simulink model "hydrocracker_stage7"  (R2025a)
settings: Solver=VariableStepAuto  StartTime=0.0  StopTime=1000  RelTol=1e-3
values from neighbouring files (symbols this model uses):
  A = 5    [hydrocracking.m]
  alpha = 0.5    [hydrocracking.m]
  alpha_r2 = 1.0    (= 1)    [hydrocracking.m]
  CH0 = 1000    [hydrocracking.m]
  CL0 = 0    [hydrocracking.m]
  CM0 = 0    [hydrocracking.m]
  dHrxn = -8e4    (= -80000)    [hydrocracking.m]
  Ea = 8e4    (= 80000)    [hydrocracking.m]
  F_H2in = 0.5    [hydrocracking.m]
  k0 = 1e6    (= 1000000)    [hydrocracking.m]
  nH2_0 = Pset * V_gas / (R*T0)    (= 2.00465078983)    [hydrocracking.m]
  Pset = 1e5    (= 100000)    [hydrocracking.m]
  R = 8.314    [hydrocracking.m]
  rhoCp = 4.0e6    (= 4000000)    [hydrocracking.m]
  T0 = 600    [hydrocracking.m]
  T_cool = 550    [hydrocracking.m]
  tau = 0.5    [hydrocracking.m]
  Tset = 600    [hydrocracking.m]
  U = 500    [hydrocracking.m]
  V_gas = 0.1    [hydrocracking.m]
  V_liq = 1.0    (= 1)    [hydrocracking.m]
libraries: slpidlib x2
settings Model: Creator=brown  LastModifiedBy=brown

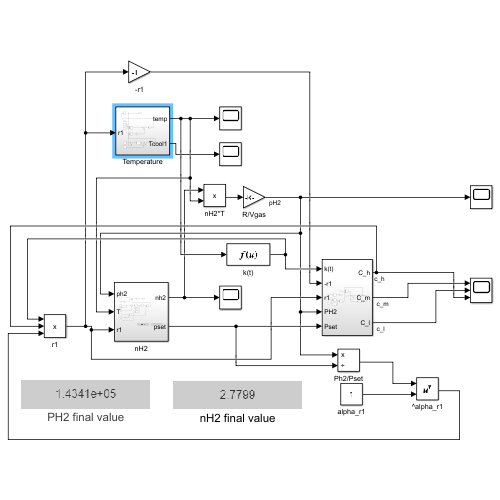
[thumbnail: Simulink's stored preview of the top-level diagram]
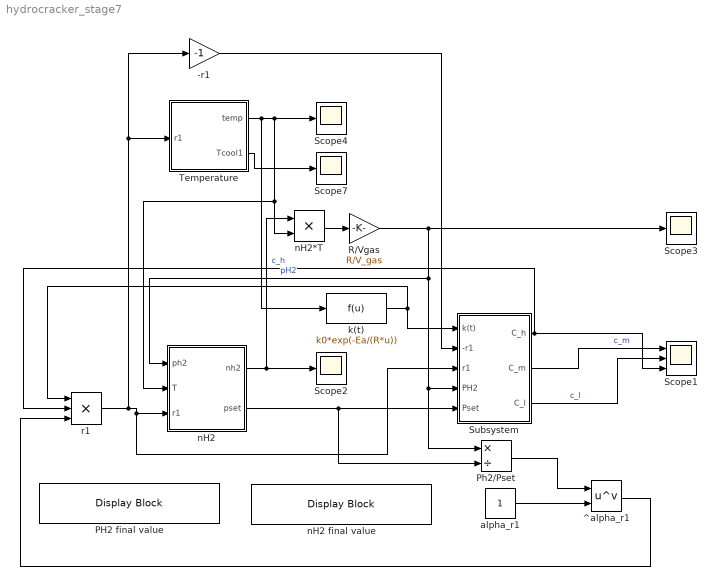
== system hydrocracker_stage7 ==
  -r1 : Gain  Gain=-1
  PH2 final value : DisplayBlock  Description=PH2 final value  LabelPosition=Hide  Transparency=1  GridColor=[0.502, 0.502, 0.502]
      settings: AttributesFormatString=%<Description>
  Ph2/Pset : Product  Inputs=*/
  R/Vgas : Gain  Gain=R/V_gas
  Scope1 : Scope  NumInputPorts=3
      settings: ActiveDisplayYMinimum=-163.95249166903488  ActiveDisplayYMaximum=1598.0751597626968
  Scope{2..4,7} (4 alike) : Scope
      Scope2 settings: ActiveDisplayYMinimum=-0.89806097221704873  ActiveDisplayYMaximum=6.0019022834382847  DataLoggingVariableName=ScopeData2
      Scope3 settings: ActiveDisplayYMinimum=-14020.662869162879  ActiveDisplayYMaximum=16737.974545965073  DataLoggingVariableName=ScopeData3
      Scope4 settings: ActiveDisplayYMinimum=580.56684447993848  ActiveDisplayYMaximum=662.48239747008381  DataLoggingVariableName=ScopeData4
      Scope7 settings: ActiveDisplayYMinimum=520.31544213629388  ActiveDisplayYMaximum=544.27149165677986  DataLoggingVariableName=ScopeData7
  Subsystem : Subsystem
  Temperature : Subsystem
  ^alpha_r1 : Math  Operator=pow
  alpha_r1 : Constant
  k(t) : Fcn  Expr=k0*exp(-Ea/(R*u))
  nH2 : Subsystem
  nH2 final value : DisplayBlock  LabelPosition=Hide  Transparency=1  GridColor=[0.502, 0.502, 0.502]
  nH2*T : Product
  r1 : Product  Inputs=3
  wires:
  k(t)/1 -> r1/1, Subsystem/1(k(t))
  nH2/1(nh2) -> nH2*T/1, Scope2/1
  r1/1 -> Subsystem/3(r1), nH2/3(r1), Temperature/1(r1), -r1/1
  R/Vgas/1 -> Scope3/1, Ph2/Pset/1, Subsystem/4(PH2), nH2/1(ph2)  "pH2"
  Temperature/2(Tcool1) -> Scope7/1
  Temperature/1(temp) -> k(t)/1, nH2/2(T), nH2*T/2, Scope4/1
  -r1/1 -> Subsystem/2(-r1)
  nH2/2(pset) -> Ph2/Pset/2, Subsystem/5(Pset)
  Subsystem/1(C_h) -> Scope1/3, r1/2  "c_h"
  Subsystem/2(C_m) -> Scope1/1  "c_m"
  Subsystem/3(C_l) -> Scope1/2  "c_l"
  Ph2/Pset/1 -> ^alpha_r1/1
  alpha_r1/1 -> ^alpha_r1/2
  ^alpha_r1/1 -> r1/3
  nH2*T/1 -> R/Vgas/1

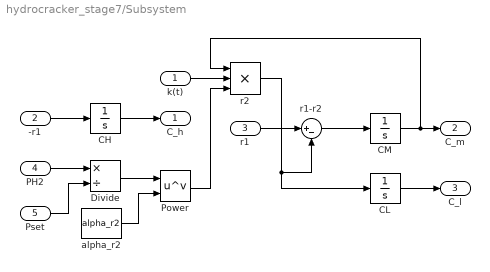
== system hydrocracker_stage7/Subsystem ==
  k(t) : Inport
  -r1 : Inport  Port=2
  r1 : Inport  Port=3
  PH2 : Inport  Port=4
  Pset : Inport  Port=5
  CH : Integrator  InitialCondition=CH0
  CL : Integrator  InitialCondition=CL0
  CM : Integrator  InitialCondition=CM0
  Divide : Product  Inputs=*/
  Power : Math  Operator=pow
  alpha_r2 : Constant  Value=alpha_r2
  r1-r2 : Sum  Inputs=|+-
  r2 : Product  Inputs=3
  C_h : Outport
  C_m : Outport  Port=2
  C_l : Outport  Port=3
  wires:
  r1/1 -> r1-r2/1
  Pset/1 -> Divide/2
  -r1/1 -> CH/1
  PH2/1 -> Divide/1
  Power/1 -> r2/3
  CM/1 -> r2/1, C_m/1
  Divide/1 -> Power/1
  CH/1 -> C_h/1
  r2/1 -> CL/1, r1-r2/2
  alpha_r2/1 -> Power/2
  k(t)/1 -> r2/2
  CL/1 -> C_l/1
  r1-r2/1 -> CM/1

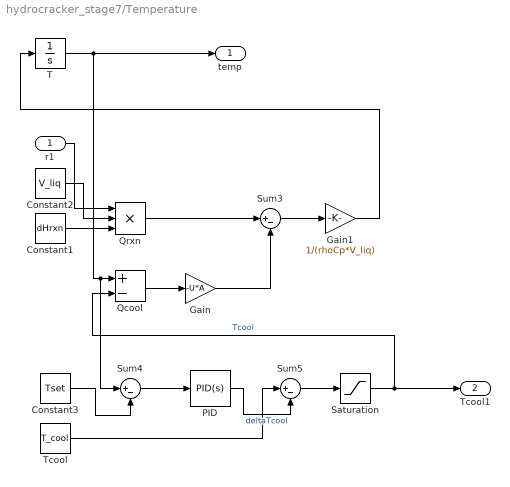
== system hydrocracker_stage7/Temperature ==
  r1 : Inport
  Constant1 : Constant  Value=dHrxn
  Constant2 : Constant  Value=V_liq
  Constant3 : Constant  Value=Tset
  Gain : Gain  Gain=-U*A
  Gain1 : Gain  Gain=1/(rhoCp*V_liq)
  PID : slpidlib/PID Controller  Controller=PID  Form=Parallel  TimeDomain=Continuous-time  UseExternalTs=off  SampleTime=-1  IntegratorMethod=Forward Euler  FilterMethod=Forward Euler  ControllerParametersSource=internal  P=0.5  I=0.001  UseKiTs=off  D=1  UseExternalDerivativeSource=off  N=100  UseFilter=on  TunerSelectOption=Transfer Function Based (PID Tuner App)  InitialConditionSource=internal  InitialConditionForIntegrator=0  InitialConditionForFilter=0  DifferentiatorICPrevScaledInput=0  ExternalReset=none  TrackingMode=off  Kt=1  LimitOutput=on  SatLimitsSource=internal  UpperSaturationLimit=inf  LowerSaturationLimit=0  LinearizeAsGain=on  AntiWindupMode=none  Kb=1  LimitIntegrator=off  UpperIntegratorSaturationLimit=inf  LowerIntegratorSaturationLimit=-inf  POutMin=[]  POutMax=[]  IOutMin=[]  IOutMax=[]  DOutMin=[]  DOutMax=[]  NOutMin=[]  NOutMax=[]  SumOutMin=[]  SumOutMax=[]  SaturationOutMin=[]  SaturationOutMax=[]  PParamMin=[]  PParamMax=[]  IParamMin=[]  IParamMax=[]  DParamMin=[]  DParamMax=[]  NParamMin=[]  NParamMax=[]  KbParamMin=[]  KbParamMax=[]  KtParamMin=[]  KtParamMax=[]  KbOutMin=[]  KbOutMax=[]  KtOutMin=[]  KtOutMax=[]  IntegratorOutMin=[]  IntegratorOutMax=[]  FilterOutMin=[]  FilterOutMax=[]  SumI1OutMin=[]  SumI1OutMax=[]  SumI2OutMin=[]  SumI2OutMax=[]  SumI3OutMin=[]  SumI3OutMax=[]  SumI4OutMin=[]  SumI4OutMax=[]  SumDOutMin=[]  SumDOutMax=[]  DifferentiatorOutMin=[]  DifferentiatorOutMax=[]  FilterDiffOutCoefMin=[]  FilterDiffOutCoefMax=[]  ReciprocalOutMin=[]  ReciprocalOutMax=[]  SumDenOutMin=[]  SumDenOutMax=[]  SumNumOutMin=[]  SumNumOutMax=[]  DivideOutMin=[]  DivideOutMax=[]  UdiffTsProdOutMin=[]  UdiffTsProdOutMax=[]  NTsProdOutMin=[]  NTsProdOutMax=[]  UintegralTsProdOutMin=[]  UintegralTsProdOutMax=[]  UngainTsProdOutMin=[]  UngainTsProdOutMax=[]  ClampingZeroOutDataTypeStr=Inherit: Inherit via back propagation  ClampingZeroOutMin=[]  ClampingZeroOutMax=[]  FilterDenConstantOutDataTypeStr=Inherit: Inherit via back propagation  FilterDenConstantOutMin=[]  FilterDenConstantOutMax=[]  PCopyOutDataTypeStr=Inherit: Inherit via back propagation  PCopyOutMin=[]  PCopyOutMax=[]  NCopyOutDataTypeStr=Inherit: Inherit via back propagation  NCopyOutMin=[]  NCopyOutMax=[]  IntegratorContinuousStateAttributes=''  IntegratorStateMustResolveToSignalObject=off  IntegratorRTWStateStorageClass=Auto  FilterContinuousStateAttributes=''  FilterStateMustResolveToSignalObject=off  FilterRTWStateStorageClass=Auto  ParallelPVariant=InternalParameters  IdealPVariant=Disabled  IVariant=InternalParameters  DVariant=InternalParameters  IntegratorVariant=Continuous  SatVariant=Enabled  AWVariant=Passthrough  PCopyVariant=Disabled  TRVariant=Disabled  FdbkBlocksVariant=Forward  IdealPFdbkVariant=Disabled  SatFdbkVariant=Disabled  DerivativeFilterVariant=ContFilter  NVariant=InternalParameters  NCopyVariant=Disabled  FilterICVariant=InternalICsFilter  IntegratorICVariant=InternalICs  ExternalResetVariant=Disabled  TRSumVariant=Passthrough  SumFdbkVariant=Disabled  SumVariant=Sum_PID  TsampFilterVariant=InternalTs  TsampNgainVariant=Passthrough  TsampIntegralVariant=Disabled_SignalSpec  ExternalSaturationOutDataTypeStr=Inherit: Same as second input  DerivativeSourceVariant=ErrorSignal  PreIntVariant=InternalPreInt
  Qcool : Sum  Inputs=+-
  Qrxn : Product  Inputs=3
  Saturation : Saturate  UpperLimit=600  LowerLimit=350
  Sum3 : Sum  Inputs=|+-
  Sum4 : Sum  Inputs=|+-
  Sum5 : Sum  Inputs=|+-
  T : Integrator  InitialCondition=T0
  Tcool : Constant  Value=T_cool
  temp : Outport
  Tcool1 : Outport  Port=2
  wires:
  Sum5/1 -> Saturation/1
  Saturation/1 -> Tcool1/1, Qcool/2  "Tcool"
  Sum3/1 -> Gain1/1
  Gain1/1 -> T/1
  Sum4/1 -> PID/1
  Constant1/1 -> Qrxn/3
  Constant2/1 -> Qrxn/2
  Tcool/1 -> Sum5/1
  Qcool/1 -> Gain/1
  Gain/1 -> Sum3/2
  PID/1 -> Sum5/2  "deltaTcool"
  Qrxn/1 -> Sum3/1
  T/1 -> Sum4/1, Qcool/1, temp/1
  r1/1 -> Qrxn/1
  Constant3/1 -> Sum4/2

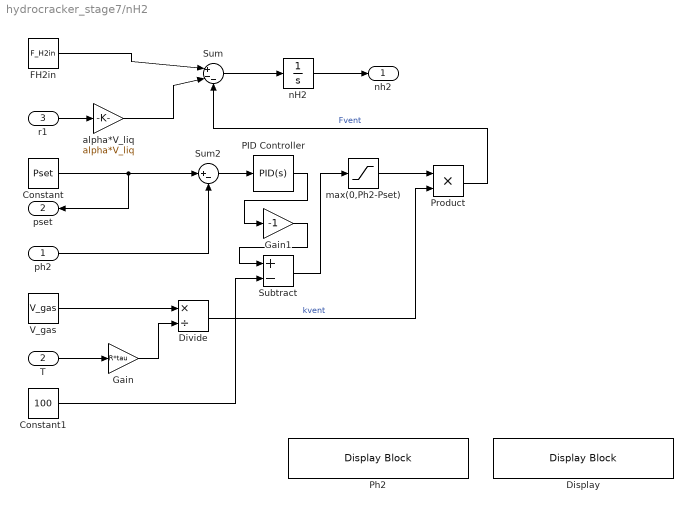
== system hydrocracker_stage7/nH2 ==
  ph2 : Inport
  T : Inport  Port=2
  r1 : Inport  Port=3
  Constant : Constant  Value=Pset
  Constant1 : Constant  Value=100
  Display : DisplayBlock  Description=Fvent  LabelPosition=Hide  Transparency=1  GridColor=[0.502, 0.502, 0.502]
      settings: AttributesFormatString=%<Description>
  Divide : Product  Inputs=*/
  FH2in : Constant  Value=F_H2in
  Gain : Gain  Gain=R*tau
  Gain1 : Gain  Gain=-1
  PID Controller : slpidlib/PID Controller  Controller=PID  Form=Parallel  TimeDomain=Continuous-time  UseExternalTs=off  SampleTime=-1  IntegratorMethod=Forward Euler  FilterMethod=Forward Euler  ControllerParametersSource=internal  P=2e-3  I=2e-4  UseKiTs=off  D=0  UseExternalDerivativeSource=off  N=100  UseFilter=on  TunerSelectOption=Transfer Function Based (PID Tuner App)  InitialConditionSource=internal  InitialConditionForIntegrator=0  InitialConditionForFilter=0  DifferentiatorICPrevScaledInput=0  ExternalReset=none  TrackingMode=off  Kt=1  LimitOutput=on  SatLimitsSource=internal  UpperSaturationLimit=inf  LowerSaturationLimit=0  LinearizeAsGain=on  AntiWindupMode=none  Kb=1  LimitIntegrator=off  UpperIntegratorSaturationLimit=inf  LowerIntegratorSaturationLimit=-inf  POutMin=[]  POutMax=[]  IOutMin=[]  IOutMax=[]  DOutMin=[]  DOutMax=[]  NOutMin=[]  NOutMax=[]  SumOutMin=[]  SumOutMax=[]  SaturationOutMin=[]  SaturationOutMax=[]  PParamMin=[]  PParamMax=[]  IParamMin=[]  IParamMax=[]  DParamMin=[]  DParamMax=[]  NParamMin=[]  NParamMax=[]  KbParamMin=[]  KbParamMax=[]  KtParamMin=[]  KtParamMax=[]  KbOutMin=[]  KbOutMax=[]  KtOutMin=[]  KtOutMax=[]  IntegratorOutMin=[]  IntegratorOutMax=[]  FilterOutMin=[]  FilterOutMax=[]  SumI1OutMin=[]  SumI1OutMax=[]  SumI2OutMin=[]  SumI2OutMax=[]  SumI3OutMin=[]  SumI3OutMax=[]  SumI4OutMin=[]  SumI4OutMax=[]  SumDOutMin=[]  SumDOutMax=[]  DifferentiatorOutMin=[]  DifferentiatorOutMax=[]  FilterDiffOutCoefMin=[]  FilterDiffOutCoefMax=[]  ReciprocalOutMin=[]  ReciprocalOutMax=[]  SumDenOutMin=[]  SumDenOutMax=[]  SumNumOutMin=[]  SumNumOutMax=[]  DivideOutMin=[]  DivideOutMax=[]  UdiffTsProdOutMin=[]  UdiffTsProdOutMax=[]  NTsProdOutMin=[]  NTsProdOutMax=[]  UintegralTsProdOutMin=[]  UintegralTsProdOutMax=[]  UngainTsProdOutMin=[]  UngainTsProdOutMax=[]  ClampingZeroOutDataTypeStr=Inherit: Inherit via back propagation  ClampingZeroOutMin=[]  ClampingZeroOutMax=[]  FilterDenConstantOutDataTypeStr=Inherit: Inherit via back propagation  FilterDenConstantOutMin=[]  FilterDenConstantOutMax=[]  PCopyOutDataTypeStr=Inherit: Inherit via back propagation  PCopyOutMin=[]  PCopyOutMax=[]  NCopyOutDataTypeStr=Inherit: Inherit via back propagation  NCopyOutMin=[]  NCopyOutMax=[]  IntegratorContinuousStateAttributes=''  IntegratorStateMustResolveToSignalObject=off  IntegratorRTWStateStorageClass=Auto  FilterContinuousStateAttributes=''  FilterStateMustResolveToSignalObject=off  FilterRTWStateStorageClass=Auto  ParallelPVariant=InternalParameters  IdealPVariant=Disabled  IVariant=InternalParameters  DVariant=InternalParameters  IntegratorVariant=Continuous  SatVariant=Enabled  AWVariant=Passthrough  PCopyVariant=Disabled  TRVariant=Disabled  FdbkBlocksVariant=Forward  IdealPFdbkVariant=Disabled  SatFdbkVariant=Disabled  DerivativeFilterVariant=ContFilter  NVariant=InternalParameters  NCopyVariant=Disabled  FilterICVariant=InternalICsFilter  IntegratorICVariant=InternalICs  ExternalResetVariant=Disabled  TRSumVariant=Passthrough  SumFdbkVariant=Disabled  SumVariant=Sum_PID  TsampFilterVariant=InternalTs  TsampNgainVariant=Passthrough  TsampIntegralVariant=Disabled_SignalSpec  ExternalSaturationOutDataTypeStr=Inherit: Same as second input  DerivativeSourceVariant=ErrorSignal  PreIntVariant=InternalPreInt
  "Ph2 " : DisplayBlock  Description=Ph2  LabelPosition=Hide  Transparency=1  GridColor=[0.502, 0.502, 0.502]
      settings: AttributesFormatString=%<Description>
  Product : Product
  Subtract : Sum  Inputs=+-
  Sum : Sum  Inputs=|+--
  Sum2 : Sum  Inputs=|+-
  V_gas : Constant  Value=V_gas
  alpha*V_liq : Gain  Gain=alpha*V_liq
  max(0,Ph2-Pset) : Saturate  UpperLimit=inf  LowerLimit=0
  nH2 : Integrator  InitialCondition=nH2_0  LimitOutput=on  LowerSaturationLimit=0
  nh2 : Outport
  pset : Outport  Port=2
  wires:
  Sum/1 -> nH2/1
  FH2in/1 -> Sum/1
  alpha*V_liq/1 -> Sum/2
  Sum2/1 -> PID Controller/1
  Constant/1 -> pset/1, Sum2/1
  r1/1 -> alpha*V_liq/1
  nH2/1 -> nh2/1
  T/1 -> Gain/1
  V_gas/1 -> Divide/1
  Gain/1 -> Divide/2
  max(0,Ph2-Pset)/1 -> Product/1
  Divide/1 -> Product/2  "kvent"
  Product/1 -> Sum/3  "Fvent"
  ph2/1 -> Sum2/2
  Constant1/1 -> Subtract/2
  Subtract/1 -> max(0,Ph2-Pset)/1
  PID Controller/1 -> Gain1/1
  Gain1/1 -> Subtract/1
